simulink model "untitled"  (R2025a)
settings: Solver=VariableStepAuto  StartTime=0.0  StopTime=50  RelTol=1e-3
model workspace (MAT data in the model file):
  J = 63
  K = 1
  K_E = 4.534
  K_m = 43.5
  L = 110
  R = 1.47
  U_N = 24
  b = 0.0011
  n0 = 12000
settings Model: Creator=josef  LastModifiedBy=josef

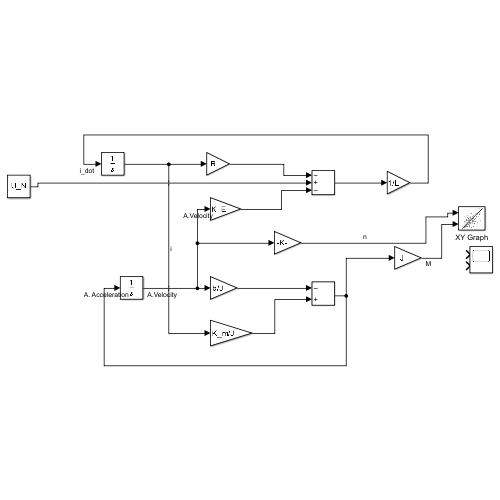
[thumbnail: Simulink's stored preview of the top-level diagram]
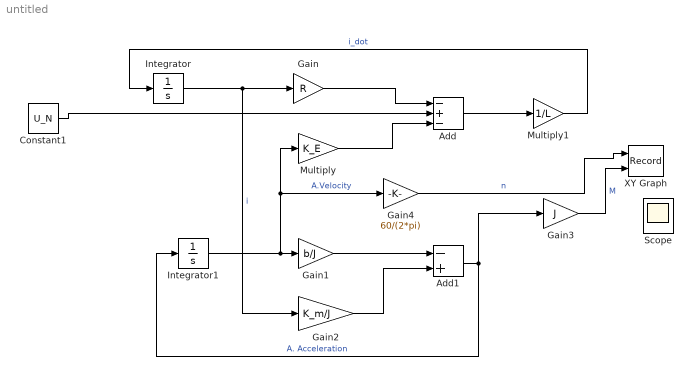
== system untitled ==
  Add : Sum  Inputs=-+-
  Add1 : Sum  Inputs=-+
  Constant1 : Constant  Value=U_N
  Gain : Gain  Gain=R
  Gain1 : Gain  Gain=b/J
  Gain2 : Gain  Gain=K_m/J
  Gain3 : Gain  Gain=J
  Gain4 : Gain  Gain=60/(2*pi)
  Integrator : Integrator
  Integrator1 : Integrator  InitialCondition=112
  Multiply : Gain  Gain=K_E
  Multiply1 : Gain  Gain=1/L
  Scope : Scope  NumInputPorts=2
      settings: ActiveDisplayYMinimum=-8.1451639951154853  ActiveDisplayYMaximum=73.306475956039378
  XY Graph : Record  NumPorts=2.0  FileSettingsInternal="{\"entries\":[{\"content\":{\"excelSettings\":{\"content\":{},\"type\":\"Streamout.ExcelSettings\"},\"parquetSettings\":{\"content\":{},\"type\":\"Streamout.ParquetSettings\"}},\"type\":\"Streamout.FileSettingStorage\",\"uuid\":\"\"}],\"packageUris\":[\"http:\\/\\/schema.mathworks.com\\/mf0\\/streamout_blocks\\/R2020a\"],\"version\":\"1.0\"}"  FrameSettings=[0, 0]  Layout=[1 1]  SignalsInternal="{\"entries\":[{\"content\":{\"signals\":[{\"content\":{\"blockPath\":[],\"dimensions\":[1],\"domain\":\"\",\"lineColor\":\"#a2142f\",\"plots\":[ 1 ],\"port\":1,\"sid\":[\"\"],\"signalID\":1,\"signalName\":\"n\"},\"type\":\"RecordBlkView.Signal\",\"uuid\":\"\"},{\"content\":{\"blockPath\":[],\"dimensions\":[1],\"domain\":\"\",\"lineColor\":\"#139fff\",\"plots\":[ 1 ],\"port\":2,\"sid\":[\"\"],\"signalID\":2,\"signalName\":\"M\"},\"type\":\"RecordBlkView.Signal\",\"uuid\":\"\"}]},\"type\":\"RecordBlkView.InputSignals\",\"uuid\":\"\"}],\"packageUris\":[\"http:\\/\\/schema.mathworks.com\\/mf0\\/streamout_blocks\\/R2020a\"],\"version\":\"1.0\"}"  VisualizationBindings="{\"xyplotplugin\":{\"info\":[{\"series\":[{\"bindingParametersList\":[{\"parameter\":\"X-Axis\",\"signalID\":1,\"signalName\":\"n\"},{\"parameter\":\"Y-Axis\",\"signalID\":2,\"signalName\":\"M\"}],\"seriesID\":0}],\"subplotID\":1}]}}"  CompatibilityTag=XY
  wires:
  Integrator/1 -> Gain/1, Gain2/1  "i"
  Multiply1/1 -> Integrator/1  "i_dot"
  Gain/1 -> Add/1
  Constant1/1 -> Add/2
  Multiply/1 -> Add/3
  Add/1 -> Multiply1/1
  Add1/1 -> Integrator1/1, Gain3/1  "A. Acceleration"
  Integrator1/1 -> Gain4/1, Multiply/1, Gain1/1  "A.Velocity"
  Gain1/1 -> Add1/1
  Gain2/1 -> Add1/2
  Gain3/1 -> XY Graph/2  "M"
  Gain4/1 -> XY Graph/1  "n"
